simulink model "LoFT_Example3"  (R2024b)
settings: Solver=ode4  StartTime=0.0  StopTime=300  FixedStep=simu.dt  RelTol=1e-3
undefined symbols (not defined in the file): body, circtime, Communication, D1, Delta, irkb, line, LoFT, p0, Pn, s, simu, trip_time, Turbwind, waves, wind
libraries: simulink x350, spsThreePhaseVIMeasurementLib x41, spsThreePhasePISectionLineLib x34, spsThreePhaseParallelRLCLoadLib x21, spsThreePhaseTransformerTwoWindingsLib x14, spsLoadFlowBusLib x10, spsThreePhaseDynamicLoadLib x9, spsSynchronousMachinepuStandardLib x7, spsExcitationSystemLib x7, spsSteamTurbineandGovernorLib x7, spsGenericPowerSystemStabilizerLib x7, spsMultiBandPowerSystemStabilizerLib x7
(part 49 of 49)

== matlab function LoFT_Example3/FOWT System/Subsystem1/FOWT4/Hydrodynamics/radiation force/MATLAB Function ==
  data: velocity input; radiationdamping output; irkb input; circtime input
function radiationdamping  = fcn(velocity,irkb,circtime)

radiationdamping  = ConvolutionIntegral_interp(velocity,irkb,circtime);
end

== matlab function LoFT_Example3/FOWT System/Subsystem5/FOWT3/Hydrodynamics/radiation force/MATLAB Function ==
  data: velocity input; radiationdamping output; irkb input; circtime input
function radiationdamping  = fcn(velocity,irkb,circtime)

radiationdamping  = ConvolutionIntegral_interp(velocity,irkb,circtime);
end

== matlab function LoFT_Example3/FOWT System/Subsystem5/FOWT4/Hydrodynamics/excitation force/WECSim Linear wave excitiation ==
  data: A input; Fext output; w input; fExtRE input; fExtIM input; phaseRand input; dw input; time input; WaveDir input; spread input; fExtMD input
function Fext = irregExcF(A,w,fExtRE,fExtIM,phaseRand,dw,time,WaveDir,spread,fExtMD)

Fext = irregExcF(A,w,fExtRE,fExtIM,phaseRand,dw,time,WaveDir,spread,fExtMD);

end

== matlab function LoFT_Example3/FOWT System/Subsystem5/FOWT4/Hydrodynamics/radiation force/MATLAB Function ==
  data: velocity input; radiationdamping output; irkb input; circtime input
function radiationdamping  = fcn(velocity,irkb,circtime)

radiationdamping  = ConvolutionIntegral_interp(velocity,irkb,circtime);
end

== matlab function LoFT_Example3/FOWT System/Subsystem5/FOWT5/Hydrodynamics/excitation force/WECSim Linear wave excitiation ==
  data: A input; Fext output; w input; fExtRE input; fExtIM input; phaseRand input; dw input; time input; WaveDir input; spread input; fExtMD input
function Fext = irregExcF(A,w,fExtRE,fExtIM,phaseRand,dw,time,WaveDir,spread,fExtMD)

Fext = irregExcF(A,w,fExtRE,fExtIM,phaseRand,dw,time,WaveDir,spread,fExtMD);

end

== matlab function LoFT_Example3/FOWT System/Subsystem5/FOWT5/Hydrodynamics/radiation force/MATLAB Function ==
  data: velocity input; radiationdamping output; irkb input; circtime input
function radiationdamping  = fcn(velocity,irkb,circtime)

radiationdamping  = ConvolutionIntegral_interp(velocity,irkb,circtime);
end

== matlab function LoFT_Example3/FOWT System/Subsystem5/FOWT6/Hydrodynamics/excitation force/WECSim Linear wave excitiation ==
  data: A input; Fext output; w input; fExtRE input; fExtIM input; phaseRand input; dw input; time input; WaveDir input; spread input; fExtMD input
function Fext = irregExcF(A,w,fExtRE,fExtIM,phaseRand,dw,time,WaveDir,spread,fExtMD)

Fext = irregExcF(A,w,fExtRE,fExtIM,phaseRand,dw,time,WaveDir,spread,fExtMD);

end

== matlab function LoFT_Example3/FOWT System/Subsystem5/FOWT6/Hydrodynamics/radiation force/MATLAB Function ==
  data: velocity input; radiationdamping output; irkb input; circtime input
function radiationdamping  = fcn(velocity,irkb,circtime)

radiationdamping  = ConvolutionIntegral_interp(velocity,irkb,circtime);
end

== matlab function LoFT_Example3/FOWT System/Subsystem1/FOWT5/Hydrodynamics/excitation force/WECSim Linear wave excitiation ==
  data: A input; Fext output; w input; fExtRE input; fExtIM input; phaseRand input; dw input; time input; WaveDir input; spread input; fExtMD input
function Fext = irregExcF(A,w,fExtRE,fExtIM,phaseRand,dw,time,WaveDir,spread,fExtMD)

Fext = irregExcF(A,w,fExtRE,fExtIM,phaseRand,dw,time,WaveDir,spread,fExtMD);

end

== matlab function LoFT_Example3/FOWT System/Subsystem5/FOWT7/Hydrodynamics/excitation force/WECSim Linear wave excitiation ==
  data: A input; Fext output; w input; fExtRE input; fExtIM input; phaseRand input; dw input; time input; WaveDir input; spread input; fExtMD input
function Fext = irregExcF(A,w,fExtRE,fExtIM,phaseRand,dw,time,WaveDir,spread,fExtMD)

Fext = irregExcF(A,w,fExtRE,fExtIM,phaseRand,dw,time,WaveDir,spread,fExtMD);

end

== matlab function LoFT_Example3/FOWT System/Subsystem5/FOWT7/Hydrodynamics/radiation force/MATLAB Function ==
  data: velocity input; radiationdamping output; irkb input; circtime input
function radiationdamping  = fcn(velocity,irkb,circtime)

radiationdamping  = ConvolutionIntegral_interp(velocity,irkb,circtime);
end

== matlab function LoFT_Example3/FOWT System/Subsystem5/FOWT8/Hydrodynamics/excitation force/WECSim Linear wave excitiation ==
  data: A input; Fext output; w input; fExtRE input; fExtIM input; phaseRand input; dw input; time input; WaveDir input; spread input; fExtMD input
function Fext = irregExcF(A,w,fExtRE,fExtIM,phaseRand,dw,time,WaveDir,spread,fExtMD)

Fext = irregExcF(A,w,fExtRE,fExtIM,phaseRand,dw,time,WaveDir,spread,fExtMD);

end

== matlab function LoFT_Example3/FOWT System/Subsystem5/FOWT8/Hydrodynamics/radiation force/MATLAB Function ==
  data: velocity input; radiationdamping output; irkb input; circtime input
function radiationdamping  = fcn(velocity,irkb,circtime)

radiationdamping  = ConvolutionIntegral_interp(velocity,irkb,circtime);
end

== matlab function LoFT_Example3/FOWT System/Subsystem5/FOWT9/Hydrodynamics/excitation force/WECSim Linear wave excitiation ==
  data: A input; Fext output; w input; fExtRE input; fExtIM input; phaseRand input; dw input; time input; WaveDir input; spread input; fExtMD input
function Fext = irregExcF(A,w,fExtRE,fExtIM,phaseRand,dw,time,WaveDir,spread,fExtMD)

Fext = irregExcF(A,w,fExtRE,fExtIM,phaseRand,dw,time,WaveDir,spread,fExtMD);

end

== matlab function LoFT_Example3/FOWT System/Subsystem5/FOWT9/Hydrodynamics/radiation force/MATLAB Function ==
  data: velocity input; radiationdamping output; irkb input; circtime input
function radiationdamping  = fcn(velocity,irkb,circtime)

radiationdamping  = ConvolutionIntegral_interp(velocity,irkb,circtime);
end

== matlab function LoFT_Example3/FOWT System/Subsystem7/FOWT1/Hydrodynamics/excitation force/WECSim Linear wave excitiation ==
  data: A input; Fext output; w input; fExtRE input; fExtIM input; phaseRand input; dw input; time input; WaveDir input; spread input; fExtMD input
function Fext = irregExcF(A,w,fExtRE,fExtIM,phaseRand,dw,time,WaveDir,spread,fExtMD)

Fext = irregExcF(A,w,fExtRE,fExtIM,phaseRand,dw,time,WaveDir,spread,fExtMD);

end
